simulink model "Qn5"  (R2022b)
settings: Solver=VariableStepAuto  StartTime=0.0  StopTime=10.0  RelTol=1e-3
settings Model: Creator=nmary  LastModifiedBy=nmary

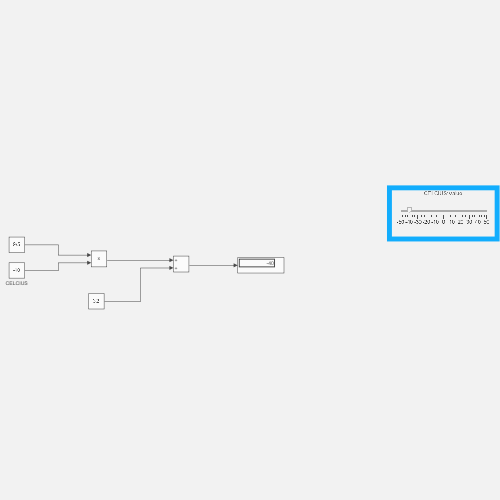
[thumbnail: Simulink's stored preview of the top-level diagram]
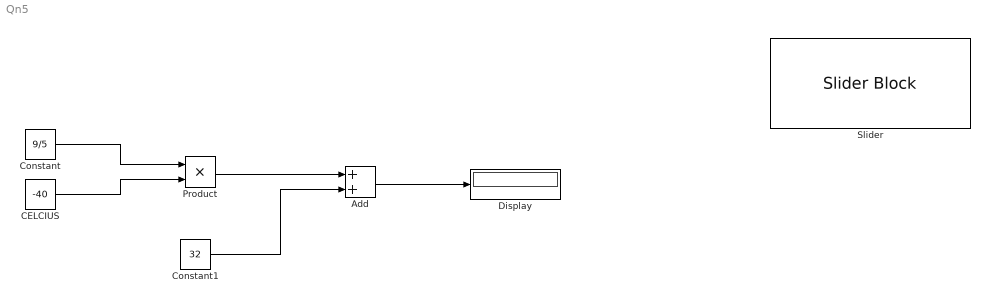
== system Qn5 ==
  Add : Sum
  CELCIUS : Constant  Value=-40
  Constant : Constant  Value=9/5
  Constant1 : Constant  Value=32
  Display : Display
  Product : Product
  Slider : SliderBlock  ScaleMin=-50  ScaleMax=50
  wires:
  CELCIUS/1 -> Product/2
  Constant/1 -> Product/1
  Product/1 -> Add/1
  Constant1/1 -> Add/2
  Add/1 -> Display/1
